simulink model "Inverter_IGBT"  (Simulink 7.5)
settings: Solver=ode45  StartTime=0.0  StopTime=.08  RelTol=1e-3
libraries: powerlib x9
settings Model: Creator=Sambhav  LastModifiedBy=Sambhav

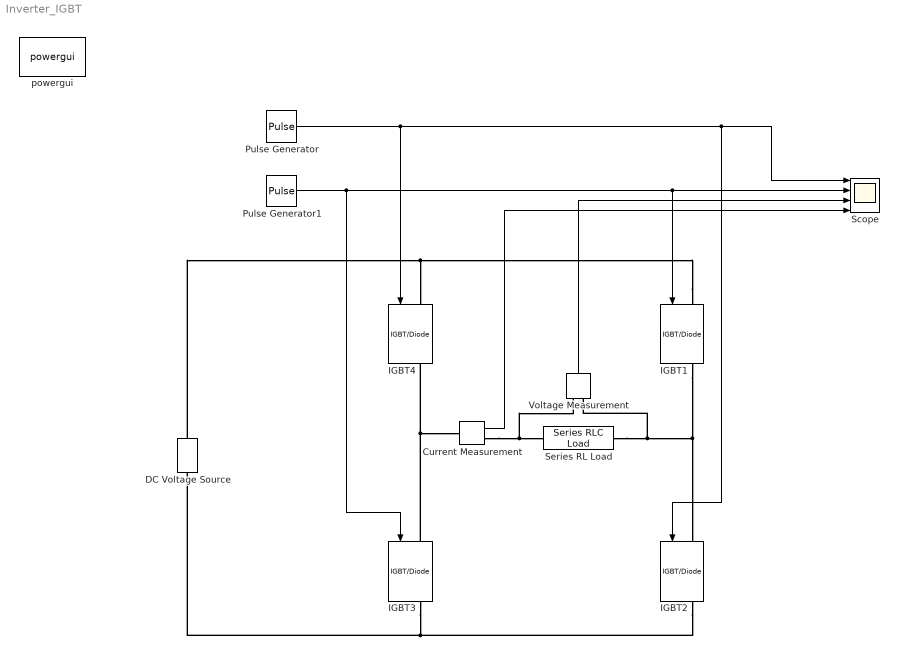
== system Inverter_IGBT ==
  Current Measurement : powerlib/Measurements/Current Measurement  DialogController=POWERSYS.PowerSysDialog  SystemSampleTime=-1  PhasorSimulation=off  OutputType=Complex  PSBequivalent=0
  DC Voltage Source : powerlib/Electrical Sources/DC Voltage Source  DialogController=POWERSYS.PowerSysDialog  SystemSampleTime=-1  Amplitude=100  Measurements=None
  IGBT{1..4} (4 alike) : powerlib/Power Electronics/IGBT//Diode  DialogController=POWERSYS.PowerSysDialog  SystemSampleTime=-1  Ron=1e-3  Rs=1e5  Cs=inf  Measurements=on
  Pulse Generator : DiscretePulseGenerator  PulseType=Time based  Amplitude=1  Period=.02  PulseWidth=50  PhaseDelay=0  SampleTime=1
  Pulse Generator1 : DiscretePulseGenerator  PulseType=Time based  Amplitude=1  Period=.02  PulseWidth=50  PhaseDelay=.01  SampleTime=1
  Scope : Scope  NumInputPorts=4
      settings: TimeRange=0.08  YMin=-0.5~-0.5~-120~-20  YMax=1.5~1.5~120~20  SampleTime=0.0001
  Series RL Load : powerlib/Elements/Series RLC Load  DialogController=POWERSYS.PowerSysDialog  PhysicalDomain=powersysdomain  SubClassName=unknown  LeftPortType=p1  RightPortType=p1  LConnTagsString=a  RConnTagsString=__new0  NominalVoltage=100  NominalFrequency=50  ActivePower=1000  InductivePower=900  CapacitivePower=0  Setx0=off  InitialVoltage=0  SetiL0=off  InitialCurrent=0  Measurements=None
  Voltage Measurement : powerlib/Measurements/Voltage Measurement  DialogController=POWERSYS.PowerSysDialog  SystemSampleTime=-1  PhasorSimulation=off  OutputType=Complex  PSBequivalent=0
  powergui : powerlib/powergui  Priority=1  SystemSampleTime=-1  SimulationMode=Continuous  SampleTime=50e-6  frequency=60  SPID=off  DisableSnubberDevices=off  DisableRonSwitches=off  DisableVfSwitches=off  SwTol=0  Interpol=off  frequencyindice=0  echomessages=off  HookPort=off  DisplayEquations=off  FunctionMessages=off  EnableUseOfTLC=off  x0status=blocks  RestoreLinks=warning  ResistiveCurrentMeasurement=off  Ylog=off  Xlog=on  ShowGrid=off  save=off  variable=ZData  ZoomFFT=off  StartTime=0.0  cycles=1  DisplayStyle=1  FreqAxis=off  MaxFrequency=1000  frequencyindicesteady=1  display=off  methode=off
  wires:
  Pulse Generator/1 -> IGBT4/1, IGBT2/1, Scope/1
  Pulse Generator1/1 -> IGBT3/1, IGBT1/1, Scope/2
  Voltage Measurement/1 -> Scope/3
  Current Measurement/1 -> Scope/4
  connections:
  IGBT1/LConn1 -- DC Voltage Source/RConn1 -- IGBT4/LConn1
  Series RL Load/RConn1 -- IGBT1/RConn1 -- IGBT2/LConn1 -- Voltage Measurement/LConn2
  IGBT3/RConn1 -- DC Voltage Source/LConn1 -- IGBT2/RConn1
  IGBT3/LConn1 -- Current Measurement/LConn1 -- IGBT4/RConn1
  Current Measurement/RConn1 -- Series RL Load/LConn1 -- Voltage Measurement/LConn1
